simulink model "Excavator_Param_BOFTOF_Setup"  (R2026a)
settings: Solver=ode45  StopTime=0.2  AbsTol=1e-3  EnableMultiTasking=on
InitFcn:
  | if(~exist('ExcvLocal'))
  | ExcvGlobal = Excavator_Pin_Locations_global('Design A');
  | ExcvLocal  = Excavator_Pin_Locations_global2local(ExcvGlobal);
  | disp('Loading default pin locations...');
  | end
undefined symbols (not defined in the file or in its folder): A1, A2, B1, B2, B3, BOFTOF_boomAngle, BOFTOF_bucketAngle, BOFTOF_stickAngle, C1, C2, C3, C4, D1, D2, excv_data, X, Y, Z
libraries: nesl_utility x36, sm_lib x29, Excavator_Parts_Param_Lib x8, Linkage_Assembly_Lib x3, Arrowhead_Lib x3
(part 1 of 2)
Description:
  | Copyright 2022-2026 The MathWorks, Inc.
settings Model: Creator=smiller  LastModifiedBy=smiller
settings SimscapeCC: SimscapeNominalValues="[{\"value\":\"1\",\"unit\":\"A\"},{\"value\":\"1\",\"unit\":\"bar\"},{\"value\":\"1\",\"unit\":\"cm^2\"},{\"value\":\"1\",\"unit\":\"cm^3/s\"},{\"value\":\"1\",\"unit\":\"kJ/kg\"},{\"value\":\"1\",\"unit\":\"kW\"},{\"value\":\"1\",\"unit\":\"l\"},{\"value\":\"1\",\"unit\":\"N\"},{\"value\":\"1\",\"unit\":\"N*m\"},{\"value\":\"1\",\"unit\":\"V\"}]"  SimscapeLogSimulationStatistics=on
settings DiagnosticsConfigSet: SimMechanicsConflictingReferenceFrames=none  SimMechanicsUnsatisfiedHighPriorityTargets=none
settings ExplorerConfigSet: InternalSimMechanicsExplorerSettings="<ExplorerConfiguration><canonicalview>default</canonicalview><AnimationSetting><BasePlaybackSpeed>1.0</BasePlaybackSpeed><PlaybackSpeedFactor>1.0</PlaybackSpeedFactor></AnimationSetting><TilePanel><TileInfo><Tiles Columns=\"1\" Count=\"1\" Rows=\"1\"><Column Weight=\"1\"/><Row Weight=\"1\"/><Tile Height=\"1\" Width=\"1\" X=\"0\" Y=\"0\"/></Tiles></TileInfo><SceneInfo><SceneViewer><BGColor><R>1</R><G>1</G><B>1</B></BGColor><Camera><DoPerspective>off</DoPerspective><Position><X>6.08452747440039499</X><Y>2.23982062543228677</Y><Z>6.37263332562871465</Z></Position><Center><X>6.08452747440039499</X><Y>2.23982062543228677</Y><Z>-1.95928139490320063e-07</Z></Center><Up><X>0</X><Y>1</Y><Z>-0</Z></Up><ViewLimDist>1</ViewLimDist><YLim>4.12210355497723135</YLim><XLim>6.50790764061927973</XLim></Camera></SceneViewer></SceneInfo></TilePanel><MechEditorPanel><Cameras/><GfxPanelCameraMap/><VideoCreator><PlaybackSpeedRatio>1.0</PlaybackSpeedRatio><FrameRate>30</FrameRate><VideoFormat>Motion JPEG AVI</VideoFormat><FrameSize>auto</FrameSize></VideoCreator></MechEditorPanel></ExplorerConfiguration>"

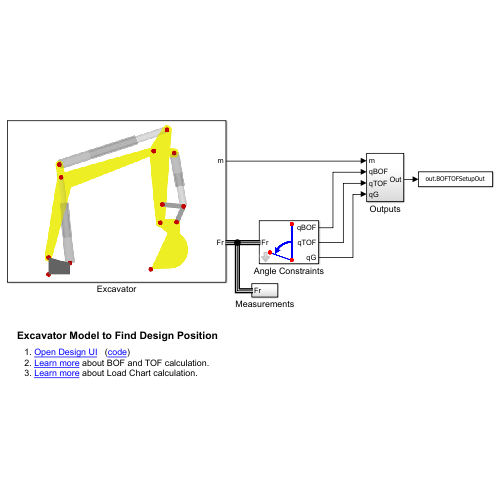
[thumbnail: Simulink's stored preview of the top-level diagram]
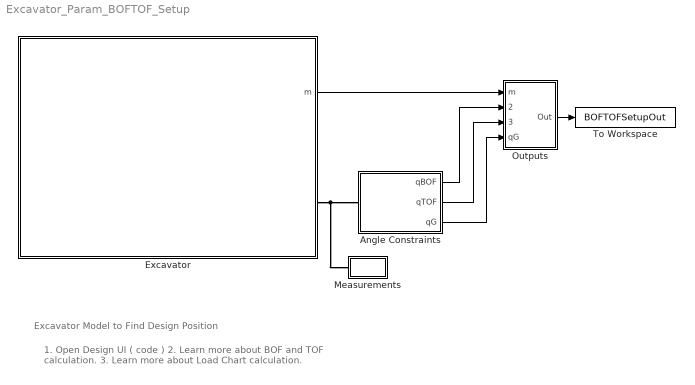
== system Excavator_Param_BOFTOF_Setup ==
  note: Excavator Model to Find Design Position
  note: 1. Open Design UI ( code )
      | 2. Learn more about BOF and TOF calculation.
      | 3. Learn more about Load Chart calculation.
  Angle Constraints : Subsystem  mask{target_angle_boom=BOFTOF_boomAngle, target_angle_stick=BOFTOF_stickAngle, target_angle_bucket=BOFTOF_bucketAngle, bar_opc=0.25, bar_dim=[2000 60 400], bar_clr=[0 0 1], checkbox_show_arc=on, arc_rad=1, arc_opc=0.25, arc_irs=0.75, arc_dep=1, arc_clr=[0 0 1]}
      mask prompts: target_angle_boom "Boom Target Angle (deg)"; target_angle_stick "Stick Target Angle (deg)"; target_angle_bucket "Bucket Target Angle (deg)"; bar_opc "Bar Opacity (0-1)"; bar_dim "Bar Dimensions [len wid depth] (m)"; bar_clr "Bar Color (0-1) [R G B]"; checkbox_show_arc "Show Arc"; arc_rad "Arc Outer Radius (m)"; arc_opc "Arc Opacity (0-1)"; arc_irs "Arc Inner Radius Scale (0-1)"; arc_dep "Arc Depth"; arc_clr "Arc Color (0-1) [R G B]"
      mask TypeOptions target_angle_boom: Boom Angle/target_angle
      mask TypeOptions target_angle_stick: Stick Angle/target_angle
      mask TypeOptions target_angle_bucket: Bucket Angle/target_angle
      mask TypeOptions bar_opc: Boom Angle/bar_opc | Bucket Angle/bar_opc | Stick Angle/bar_opc
      mask TypeOptions bar_dim: Boom Angle/bar_dim | Bucket Angle/bar_dim | Stick Angle/bar_dim
      mask TypeOptions bar_clr: Boom Angle/bar_clr | Bucket Angle/bar_clr | Stick Angle/bar_clr
      mask TypeOptions checkbox_show_arc: Boom Angle/checkbox_show_arc | Bucket Angle/checkbox_show_arc | Stick Angle/checkbox_show_arc
      mask TypeOptions arc_rad: Boom Angle/arc_rad | Bucket Angle/arc_rad | Stick Angle/arc_rad
      mask TypeOptions arc_opc: Boom Angle/arc_opc | Bucket Angle/arc_opc | Stick Angle/arc_opc
      mask TypeOptions arc_irs: Boom Angle/arc_irs | Bucket Angle/arc_irs | Stick Angle/arc_irs
      mask TypeOptions arc_dep: Boom Angle/arc_dep | Bucket Angle/arc_dep | Stick Angle/arc_dep
      mask TypeOptions arc_clr: Boom Angle/arc_clr | Bucket Angle/arc_clr | Stick Angle/arc_clr
      mask DialogControl Container3 Prompt: Appearance
      mask Display: image('Angle_Tools_IMAGE.png')
  Excavator : Subsystem
      mask Display: image('Excavator_Param_Full_IMAGE.png');
  Measurements : Subsystem
  Outputs : Subsystem
  To Workspace : ToWorkspace  VariableName=BOFTOFSetupOut  SaveFormat=Timeseries  SampleTime=-1
  wires:
  Outputs/1(Out) -> To Workspace/1
  Angle Constraints/1(qBOF) -> Outputs/2(qBOF)
  Angle Constraints/2(qTOF) -> Outputs/3(qTOF)
  Excavator/1(m) -> Outputs/1(m)
  Angle Constraints/3(qG) -> Outputs/4(qG)
  connections:
  Excavator/RConn1 -- Measurements/LConn1 -- Angle Constraints/LConn1

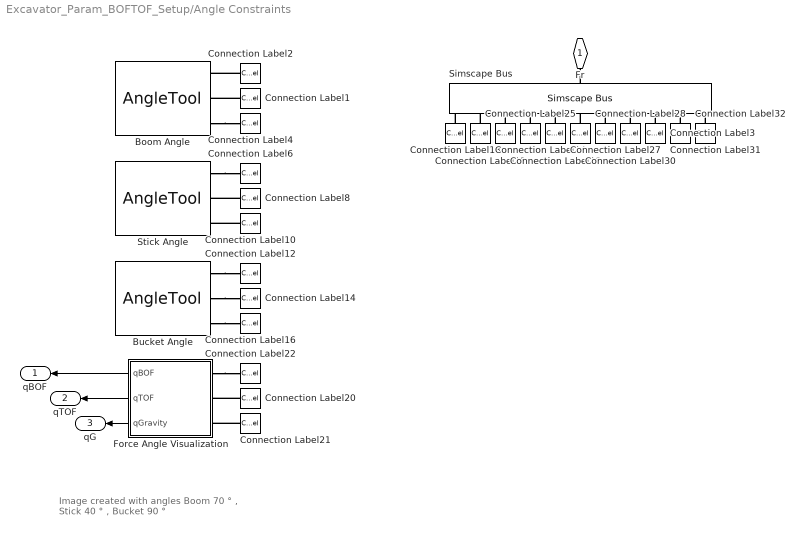
== system Excavator_Param_BOFTOF_Setup/Angle Constraints ==
  note: Image created with angles
      | Boom 70 ° , Stick 40 ° , Bucket 90 °
  Boom Angle : Linkage_Assembly_Lib/AngleTool  target_angle=target_angle_boom  checkbox_show_arc=on  arc_irs=arc_irs  arc_dep=arc_dep  arc_rad=arc_rad  arc_opc=arc_opc  arc_clr=arc_clr  bar_dim=bar_dim  bar_opc=bar_opc  bar_clr=bar_clr
  Bucket Angle : Linkage_Assembly_Lib/AngleTool  target_angle=target_angle_bucket  checkbox_show_arc=on  arc_irs=arc_irs  arc_dep=arc_dep  arc_rad=arc_rad  arc_opc=arc_opc  arc_clr=arc_clr  bar_dim=bar_dim  bar_opc=bar_opc  bar_clr=bar_clr
  Connection Label1 : ConnectionLabel  Label=A1
  Connection Label10 : ConnectionLabel  Label=B2
  Connection Label12 : ConnectionLabel  Label=D1
  Connection Label14 : ConnectionLabel  Label=C4
  Connection Label16 : ConnectionLabel  Label=C2
  Connection Label18 : ConnectionLabel  Label=A1
  Connection Label19 : ConnectionLabel  Label=A2
  Connection Label2 : ConnectionLabel  Label=A2
  Connection Label20 : ConnectionLabel  Label=C4
  Connection Label21 : ConnectionLabel  Label=B3
  Connection Label22 : ConnectionLabel  Label=D2
  Connection Label24 : ConnectionLabel  Label=B1
  Connection Label25 : ConnectionLabel  Label=B2
  Connection Label26 : ConnectionLabel  Label=B3
  Connection Label27 : ConnectionLabel  Label=C1
  Connection Label28 : ConnectionLabel  Label=C2
  Connection Label3 : ConnectionLabel  Label=C4
  Connection Label30 : ConnectionLabel  Label=C3
  Connection Label31 : ConnectionLabel  Label=D1
  Connection Label32 : ConnectionLabel  Label=D2
  Connection Label4 : ConnectionLabel  Label=B1
  Connection Label6 : ConnectionLabel  Label=C1
  Connection Label8 : ConnectionLabel  Label=B3
  Force Angle Visualization : Subsystem
      mask Display: image('Arrow_with_Reference_Line_IMAGE.png')
  Simscape Bus : SimscapeBus  HierarchyStrings=A1;A2;B1;B2;B3;C1;C2;C3;C4;D1;D2
  Stick Angle : Linkage_Assembly_Lib/AngleTool  target_angle=target_angle_stick  checkbox_show_arc=on  arc_irs=arc_irs  arc_dep=arc_dep  arc_rad=arc_rad  arc_opc=arc_opc  arc_clr=arc_clr  bar_dim=bar_dim  bar_opc=bar_opc  bar_clr=bar_clr
  Fr : PMIOPort  Side=Left
  qBOF : Outport
  qTOF : Outport  Port=2
  qG : Outport  Port=3
  wires:
  Force Angle Visualization/2(qTOF) -> qTOF/1
  Force Angle Visualization/1(qBOF) -> qBOF/1
  Force Angle Visualization/3(qGravity) -> qG/1
  connections:
  Connection Label10/LConn1 -- Stick Angle/LConn3
  Bucket Angle/LConn1 -- Connection Label12/LConn1
  Stick Angle/LConn1 -- Connection Label6/LConn1
  Boom Angle/LConn3 -- Connection Label4/LConn1
  Connection Label1/LConn1 -- Boom Angle/LConn2
  Connection Label21/LConn1 -- Force Angle Visualization/LConn3
  Connection Label2/LConn1 -- Boom Angle/LConn1
  Simscape Bus/RConn1 -- Fr/RConn1
  Connection Label8/LConn1 -- Stick Angle/LConn2
  Bucket Angle/LConn3 -- Connection Label16/LConn1
  Bucket Angle/LConn2 -- Connection Label14/LConn1
  Force Angle Visualization/LConn1 -- Connection Label22/LConn1
  Connection Label20/LConn1 -- Force Angle Visualization/LConn2
  Connection Label31/LConn1 -- Simscape Bus/LConn10
  Connection Label24/LConn1 -- Simscape Bus/LConn3
  Connection Label27/LConn1 -- Simscape Bus/LConn6
  Connection Label28/LConn1 -- Simscape Bus/LConn7
  Connection Label25/LConn1 -- Simscape Bus/LConn4
  Connection Label32/LConn1 -- Simscape Bus/LConn11
  Connection Label3/LConn1 -- Simscape Bus/LConn9
  Connection Label30/LConn1 -- Simscape Bus/LConn8
  Connection Label19/LConn1 -- Simscape Bus/LConn2
  Connection Label26/LConn1 -- Simscape Bus/LConn5
  Connection Label18/LConn1 -- Simscape Bus/LConn1

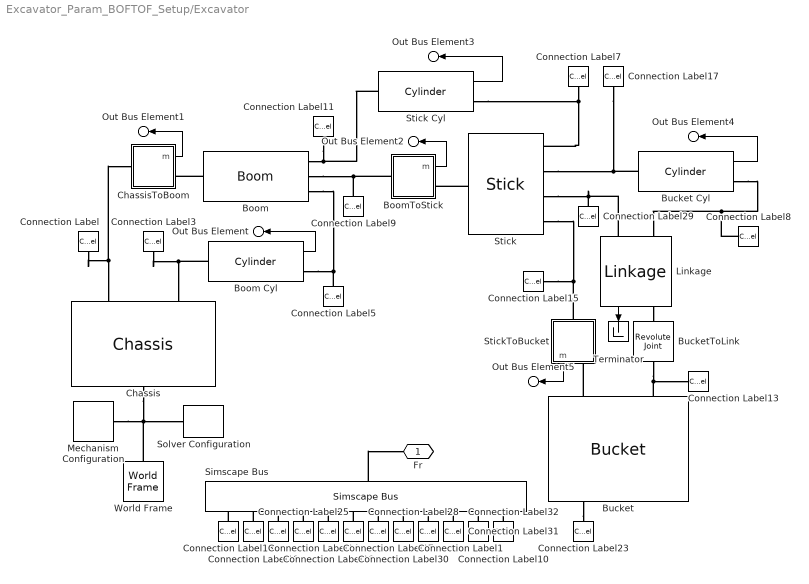
== system Excavator_Param_BOFTOF_Setup/Excavator ==
  Boom : Excavator_Parts_Param_Lib/Boom  part_thk=excv_data.arm.thk*1.05  part_clr=excv_data.arm.clr  opc=excv_data.arm.opc  pin_len=excv_data.pin.len  pin_rad=excv_data.pin.rad  pin_clr=excv_data.pin.clr  pin_opc=excv_data.pin.opc  Boom=ExcvLocal.Boom  part_mass=LoadChart_BoomMass
  Boom Cyl : Excavator_Parts_Param_Lib/Cylinder  cyl_clr=excv_data.cyl.clr  cyl_rad=excv_data.cyl.rad  cyl_opc=excv_data.cyl.opc  cyl_len=excv_data.boomcyl.len  pist_clr=excv_data.pist.clr  pist_rad=excv_data.pist.rad  pist_opc=excv_data.pist.opc  pist_len=excv_data.boompist.len
  BoomToStick : Subsystem
      mask Display: image('Excavator_Revolute_IMAGE.png')
  Bucket : Excavator_Parts_Param_Lib/Bucket  part_thk=excv_data.bucket.thk  part_clr=excv_data.bucket.clr  opc=excv_data.arm.opc  pin_len=excv_data.pin.len  pin_rad=excv_data.pin.rad  pin_clr=excv_data.pin.clr  pin_opc=excv_data.pin.opc  Bucket=ExcvLocal.Bucket  part_mass=LoadChart_BucketMass
  Bucket Cyl : Excavator_Parts_Param_Lib/Cylinder  cyl_clr=excv_data.cyl.clr  cyl_rad=excv_data.cyl.rad  cyl_opc=excv_data.cyl.opc  cyl_len=excv_data.bucketcyl.len  pist_clr=excv_data.pist.clr  pist_rad=excv_data.pist.rad  pist_opc=excv_data.pist.opc  pist_len=excv_data.bucketpist.len
  BucketToLink : sm_lib/Joints/Revolute Joint  JointMode=Normal  CompositeWrenchDir=FollowerOnBase  CompositeWrenchFrame=BaseFrame  SenseConstraintForce=off  SenseConstraintTorque=off  SenseTotalForce=off  SenseTotalTorque=off  PositionTargetSpecify=off  PositionTargetPriority=Low  PositionTargetValue=0  PositionTargetValueUnits=deg  VelocityTargetSpecify=off  VelocityTargetPriority=High  VelocityTargetValue=0  VelocityTargetValueUnits=deg/s  EquilibriumPosition=0  EquilibriumPositionUnits=deg  SpringStiffness=0  SpringStiffnessUnits=N*m/deg  DampingCoefficient=0  DampingCoefficientUnits=N*m/(deg/s)  LowerLimitSpecify=off  LowerLimitBound=-90  LowerLimitBoundUnits=deg  LowerLimitStiffness=1e4  LowerLimitStiffnessUnits=N*m/deg  LowerLimitDamping=10  LowerLimitDampingUnits=N*m/(deg/s)  LowerLimitTransitionRegionWidth=0.1  LowerLimitTransitionRegionWidthUnits=deg  UpperLimitSpecify=off  UpperLimitBound=90  UpperLimitBoundUnits=deg  UpperLimitStiffness=1e4  UpperLimitStiffnessUnits=N*m/deg  UpperLimitDamping=10  UpperLimitDampingUnits=N*m/(deg/s)  UpperLimitTransitionRegionWidth=0.1  UpperLimitTransitionRegionWidthUnits=deg  TorqueActuationMode=NoTorque  MotionActuationMode=ComputedMotion  SensePosition=off  SenseVelocity=off  SenseAcceleration=off  SenseTorqueForce=off  SenseLowerLimitTorqueForce=off  SenseUpperLimitTorqueForce=off
  Chassis : Excavator_Parts_Param_Lib/Chassis  Chassis=ExcvLocal.Chassis  opc=0  part_thk=excv_data.chassis.thk  part_clr=excv_data.chassis.clr  pin_clr=excv_data.pin.clr  pin_rad=excv_data.pin.rad  pin_len=excv_data.pin.len  pin_opc=excv_data.pin.opc
  ChassisToBoom : Subsystem
      mask Display: image('Excavator_Revolute_IMAGE.png')
  Connection Label : ConnectionLabel  Label=A1
  Connection Label1 : ConnectionLabel  Label=C4
  Connection Label10 : ConnectionLabel  Label=E1
  Connection Label11 : ConnectionLabel  Label=B2
  Connection Label13 : ConnectionLabel  Label=D1
  Connection Label15 : ConnectionLabel  Label=C4
  Connection Label17 : ConnectionLabel  Label=C2
  Connection Label18 : ConnectionLabel  Label=A1
  Connection Label19 : ConnectionLabel  Label=A2
  Connection Label23 : ConnectionLabel  Label=D2
  Connection Label24 : ConnectionLabel  Label=B1
  Connection Label25 : ConnectionLabel  Label=B2
  Connection Label26 : ConnectionLabel  Label=B3
  Connection Label27 : ConnectionLabel  Label=C1
  Connection Label28 : ConnectionLabel  Label=C2
  Connection Label29 : ConnectionLabel  Label=C3
  Connection Label3 : ConnectionLabel  Label=A2
  Connection Label30 : ConnectionLabel  Label=C3
  Connection Label31 : ConnectionLabel  Label=D1
  Connection Label32 : ConnectionLabel  Label=D2
  Connection Label5 : ConnectionLabel  Label=B1
  Connection Label7 : ConnectionLabel  Label=C1
  Connection Label8 : ConnectionLabel  Label=E1
  Connection Label9 : ConnectionLabel  Label=B3
  Linkage : Excavator_Parts_Param_Lib/Linkage  Linkage=ExcvLocal.Linkage  link_clr=excv_data.link.clr  link_thk=excv_data.link.thk  opc=excv_data.link.opc  pin_clr=excv_data.pin.clr  pin_rad=excv_data.pin.rad  pin_len=excv_data.pin.len  pin_opc=excv_data.pin.opc
  Mechanism Configuration : sm_lib/Utilities/Mechanism Configuration  UniformGravity=Constant  GravityVector=[0 -9.80665 0]  GravityVectorUnits=m/s^2  LinearizationDelta=0.001  JointModeTransitionNonlinearIterations=2
  Simscape Bus : SimscapeBus  HierarchyStrings=A1;A2;B1;B2;B3;C1;C2;C3;C4;D1;D2;E1
  Solver Configuration : nesl_utility/Solver Configuration  PhysicalDomain=network_engine_domain  SubClassName=solver  LeftPortType=input  RightPortType=generic  Tones=[]  Harmonics=[]  SimulateNoise=off  Profile=off  UseLocalSampling=off  EnableSwitchedLinearOptims=on  FrequencyDomain=off  UseCCode=off  RelTol=0.001  AbsTol=1e-06  MinStep=1e-09  ToWorkspace=off  RevertToSquareIcSolve=off  NumHomotopyIterations=100  PhasorMode=off  PhasorModeNumHarmonics=1  ConsistencySolver=NEWTON_FTOL  CanonicalOrdering=UNORDERED  OptimizeIntermediates=UNOPTIMIZED  IndexReductionMethod=DerivativeReplacement  DoDC=off  ResidualTolerance=1e-09  ConsistencyTolSource=GLOBAL  ConsistencyAbsTol=0.001  ConsistencyRelTol=0.001  ConsistencyTolFactor=0.001  UseLocalSolver=off  LocalSolverChoice=NE_BACKWARD_EULER_ADVANCER  ResolveIndetEquations=on  FunctionEvalNumThread=1  LocalSolverSampleTime=0.001  DoFixedCost=off  MaxNonlinIter=3  MaxModeIter=2  ComputeImpulses=off  ImpulseIterations=2  LinearAlgebra=Sparse  LinearAlgebraNumThread=0  EquationFormulation=NE_TIME_EF  DelaysMemoryBudget=1024  AutomaticFiltering=on  FilteringTimeConstant=0.001  PartitionStorageMethod=AS_NEEDED  PartitionMemoryBudget=1024  PartitionMethod=FAST  MultibodyUseLocalSolver=off  MultibodyLocalSolverChoice=ODE1  MultibodyLocalSolverSampleTime=0.001
  Stick : Excavator_Parts_Param_Lib/Stick  part_thk=excv_data.arm.thk  part_clr=excv_data.arm.clr*0.9  opc=excv_data.arm.opc  pin_len=excv_data.pin.len  pin_rad=excv_data.pin.rad  pin_opc=excv_data.pin.opc  pin_clr=excv_data.pin.clr  Stick=ExcvLocal.Stick  part_mass=LoadChart_StickMass
  Stick Cyl : Excavator_Parts_Param_Lib/Cylinder  cyl_clr=excv_data.cyl.clr  cyl_rad=excv_data.cyl.rad  cyl_opc=excv_data.cyl.opc  cyl_len=excv_data.stickcyl.len  pist_clr=excv_data.pist.clr  pist_rad=excv_data.pist.rad  pist_opc=excv_data.pist.opc  pist_len=excv_data.stickpist.len
  StickToBucket : Subsystem
      mask Display: image('Excavator_Revolute_IMAGE.png')
  Terminator : Terminator
  World Frame : sm_lib/Frames and Transforms/World Frame
  Fr : PMIOPort  Side=Right
  Out Bus Element : Outport  PortName=m  Element=cBoomL
  Out Bus Element3 : Outport  PortName=m  Element=cStick
  Out Bus Element4 : Outport  PortName=m  Element=cBucket
  Out Bus Element1 : Outport  PortName=m  Element=jC2B
  Out Bus Element2 : Outport  PortName=m  Element=jB2S
  Out Bus Element5 : Outport  PortName=m  Element=jS2B
  wires:
  Boom Cyl/1 -> Out Bus Element/1
  Stick Cyl/1 -> Out Bus Element3/1
  Bucket Cyl/1 -> Out Bus Element4/1
  ChassisToBoom/1(m) -> Out Bus Element1/1
  BoomToStick/1(m) -> Out Bus Element2/1
  StickToBucket/1(m) -> Out Bus Element5/1
  Linkage/1 -> Terminator/1
  connections:
  Connection Label/LConn1 -- Chassis/RConn1 -- ChassisToBoom/LConn1
  Connection Label29/LConn1 -- Stick/RConn3 -- Linkage/LConn1
  Connection Label7/LConn1 -- Stick Cyl/RConn1 -- Stick/RConn1
  Connection Label11/LConn1 -- Boom/RConn1 -- Stick Cyl/LConn1
  Bucket/LConn1 -- StickToBucket/RConn1
  Connection Label5/LConn1 -- Boom Cyl/RConn1 -- Boom/RConn3
  World Frame/RConn1 -- Chassis/LConn1 -- Solver Configuration/RConn1 -- Mechanism Configuration/RConn1
  BucketToLink/LConn1 -- Bucket/LConn2 -- Connection Label13/LConn1
  Connection Label17/LConn1 -- Bucket Cyl/LConn1 -- Stick/RConn2
  Simscape Bus/RConn1 -- Fr/RConn1
  Connection Label3/LConn1 -- Boom Cyl/LConn1 -- Chassis/RConn2
  Boom/LConn1 -- ChassisToBoom/RConn1
  Connection Label9/LConn1 -- Boom/RConn2 -- BoomToStick/LConn1
  Stick/LConn1 -- BoomToStick/RConn1
  StickToBucket/LConn1 -- Stick/RConn4 -- Connection Label15/LConn1
  Bucket/RConn1 -- Connection Label23/LConn1
  Bucket Cyl/RConn1 -- Connection Label8/LConn1 -- Linkage/LConn2
  Linkage/RConn1 -- BucketToLink/RConn1
  Connection Label26/LConn1 -- Simscape Bus/LConn5
  Connection Label25/LConn1 -- Simscape Bus/LConn4
  Connection Label28/LConn1 -- Simscape Bus/LConn7
  Connection Label24/LConn1 -- Simscape Bus/LConn3
  Connection Label31/LConn1 -- Simscape Bus/LConn10
  Connection Label1/LConn1 -- Simscape Bus/LConn9
  Connection Label19/LConn1 -- Simscape Bus/LConn2
  Connection Label30/LConn1 -- Simscape Bus/LConn8
  Connection Label27/LConn1 -- Simscape Bus/LConn6
  Connection Label18/LConn1 -- Simscape Bus/LConn1
  Connection Label32/LConn1 -- Simscape Bus/LConn11
  Connection Label10/LConn1 -- Simscape Bus/LConn12

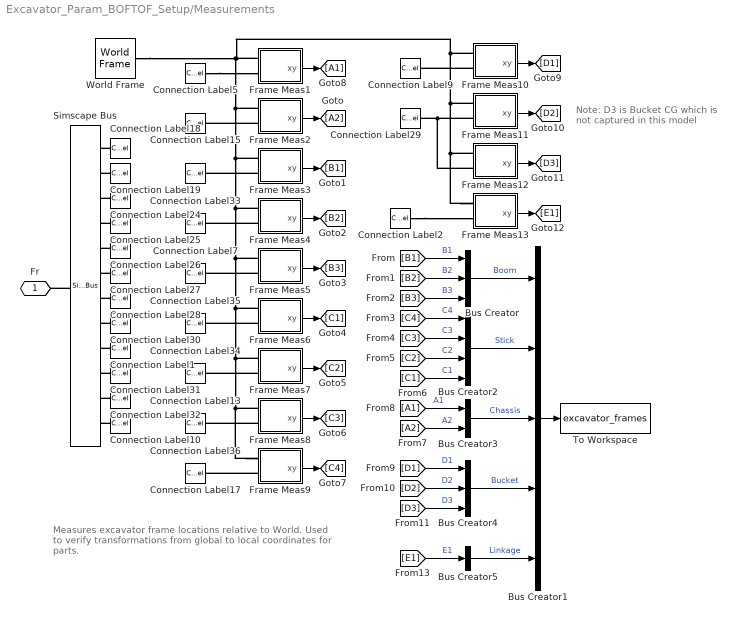
== system Excavator_Param_BOFTOF_Setup/Measurements ==
  note: Measures excavator frame locations relative to World. Used to verify transformations from global to local coordinates for parts.
  note: Note: D3 is Bucket CG which is not captured in this model
  Bus Creator : BusCreator  Inputs=3
  Bus Creator1 : BusCreator  Inputs=5
  Bus Creator2 : BusCreator  Inputs=4
  Bus Creator3 : BusCreator  Inputs=2
  Bus Creator4 : BusCreator  Inputs=3
  Bus Creator5 : BusCreator  Inputs=1
  Connection Label1 : ConnectionLabel  Label=C4
  Connection Label10 : ConnectionLabel  Label=E1
  Connection Label13 : ConnectionLabel  Label=C2
  Connection Label15 : ConnectionLabel  Label=A2
  Connection Label17 : ConnectionLabel  Label=C4
  Connection Label18 : ConnectionLabel  Label=A1
  Connection Label19 : ConnectionLabel  Label=A2
  Connection Label2 : ConnectionLabel  Label=E1
  Connection Label24 : ConnectionLabel  Label=B1
  Connection Label25 : ConnectionLabel  Label=B2
  Connection Label26 : ConnectionLabel  Label=B3
  Connection Label27 : ConnectionLabel  Label=C1
  Connection Label28 : ConnectionLabel  Label=C2
  Connection Label29 : ConnectionLabel  Label=D2
  Connection Label30 : ConnectionLabel  Label=C3
  Connection Label31 : ConnectionLabel  Label=D1
  Connection Label32 : ConnectionLabel  Label=D2
  Connection Label33 : ConnectionLabel  Label=B1
  Connection Label34 : ConnectionLabel  Label=C1
  Connection Label35 : ConnectionLabel  Label=B3
  Connection Label36 : ConnectionLabel  Label=C3
  Connection Label5 : ConnectionLabel  Label=A1
  Connection Label7 : ConnectionLabel  Label=B2
  Connection Label9 : ConnectionLabel  Label=D1
  Frame Meas1 : Subsystem
  Frame Meas10 : Subsystem
  Frame Meas11 : Subsystem
  Frame Meas12 : Subsystem
  Frame Meas13 : Subsystem
  Frame Meas2 : Subsystem
  Frame Meas3 : Subsystem
  Frame Meas4 : Subsystem
  Frame Meas5 : Subsystem
  Frame Meas6 : Subsystem
  Frame Meas7 : Subsystem
  Frame Meas8 : Subsystem
  Frame Meas9 : Subsystem
  Simscape Bus : SimscapeBus  HierarchyStrings=A1;A2;B1;B2;B3;C1;C2;C3;C4;D1;D2;E1
  To Workspace : ToWorkspace  VariableName=excavator_frames  SaveFormat=Timeseries  SampleTime=-1
      settings: MaxDataPoints=1
  World Frame : sm_lib/Frames and Transforms/World Frame
  Fr : PMIOPort  Side=Left
  wires:
  Frame Meas13/1(xy) -> [E1]
  [B3] -> Bus Creator/3  "B3"
  Frame Meas10/1(xy) -> [D1]
  Frame Meas9/1(xy) -> [C4]
  [A2] -> Bus Creator3/2  "A2"
  Frame Meas12/1(xy) -> [D3]
  Frame Meas2/1(xy) -> [A2]
  Frame Meas6/1(xy) -> [C1]
  [B2] -> Bus Creator/2  "B2"
  Frame Meas3/1(xy) -> [B1]
  Frame Meas5/1(xy) -> [B3]
  [C3] -> Bus Creator2/2  "C3"
  [A1] -> Bus Creator3/1  "A1"
  Frame Meas4/1(xy) -> [B2]
  Frame Meas1/1(xy) -> [A1]
  [D3] -> Bus Creator4/3  "D3"
  Bus Creator/1 -> Bus Creator1/1  "Boom"
  [B1] -> Bus Creator/1  "B1"
  Frame Meas8/1(xy) -> [C3]
  [D1] -> Bus Creator4/1  "D1"
  Frame Meas11/1(xy) -> [D2]
  Frame Meas7/1(xy) -> [C2]
  Bus Creator3/1 -> Bus Creator1/3  "Chassis"
  [C1] -> Bus Creator2/4  "C1"
  [C2] -> Bus Creator2/3  "C2"
  Bus Creator4/1 -> Bus Creator1/4  "Bucket"
  [D2] -> Bus Creator4/2  "D2"
  Bus Creator2/1 -> Bus Creator1/2  "Stick"
  [E1] -> Bus Creator5/1  "E1"
  Bus Creator1/1 -> To Workspace/1
  [C4] -> Bus Creator2/1  "C4"
  Bus Creator5/1 -> Bus Creator1/5  "Linkage"
  connections:
  Frame Meas13/LConn1 -- Frame Meas12/LConn1 -- Frame Meas11/LConn1 -- Frame Meas10/LConn1 -- Frame Meas1/LConn1 -- World Frame/RConn1 -- Frame Meas2/LConn1 -- Frame Meas3/LConn1 -- Frame Meas4/LConn1 -- Frame Meas5/LConn1 -- Frame Meas6/LConn1 -- Frame Meas9/LConn1 -- Frame Meas8/LConn1 -- Frame Meas7/LConn1
  Connection Label5/LConn1 -- Frame Meas1/LConn2
  Connection Label2/LConn1 -- Frame Meas13/LConn2
  Frame Meas10/LConn2 -- Connection Label9/LConn1
  Frame Meas7/LConn2 -- Connection Label13/LConn1
  Frame Meas9/LConn2 -- Connection Label17/LConn1
  Frame Meas8/LConn2 -- Connection Label36/LConn1
  Frame Meas4/LConn2 -- Connection Label7/LConn1
  Frame Meas11/LConn2 -- Frame Meas12/LConn2 -- Connection Label29/LConn1
  Frame Meas6/LConn2 -- Connection Label34/LConn1
  Frame Meas3/LConn2 -- Connection Label33/LConn1
  Frame Meas5/LConn2 -- Connection Label35/LConn1
  Frame Meas2/LConn2 -- Connection Label15/LConn1
  Simscape Bus/RConn1 -- Fr/RConn1
  Connection Label32/LConn1 -- Simscape Bus/LConn11
  Connection Label30/LConn1 -- Simscape Bus/LConn8
  Connection Label1/LConn1 -- Simscape Bus/LConn9
  Connection Label19/LConn1 -- Simscape Bus/LConn2
  Connection Label27/LConn1 -- Simscape Bus/LConn6
  Connection Label31/LConn1 -- Simscape Bus/LConn10
  Connection Label25/LConn1 -- Simscape Bus/LConn4
  Connection Label18/LConn1 -- Simscape Bus/LConn1
  Connection Label28/LConn1 -- Simscape Bus/LConn7
  Connection Label26/LConn1 -- Simscape Bus/LConn5
  Connection Label10/LConn1 -- Simscape Bus/LConn12
  Connection Label24/LConn1 -- Simscape Bus/LConn3

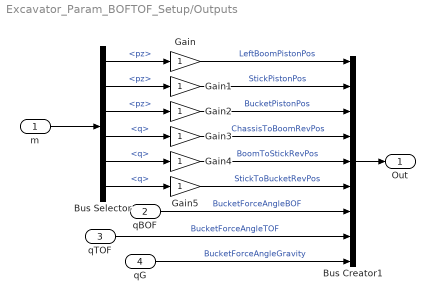
== system Excavator_Param_BOFTOF_Setup/Outputs ==
  m : Inport
  qBOF : Inport  Port=2
  qTOF : Inport  Port=3
  qG : Inport  Port=4
  Bus Creator1 : BusCreator  Inputs=9
  Bus Selector : BusSelector  OutputSignals=cBoomL.pz,cStick.pz,cBucket.pz,jC2B.q,jB2S.q,jS2B.q
  Gain{,1..5} (6 alike) : Gain
  Out : Outport
  wires:
  Gain5/1 -> Bus Creator1/6  "StickToBucketRevPos"
  Bus Selector/2 -> Gain1/1  "<pz>"
  Bus Selector/1 -> Gain/1  "<pz>"
  Gain1/1 -> Bus Creator1/2  "StickPistonPos"
  Bus Selector/4 -> Gain3/1  "<q>"
  Gain/1 -> Bus Creator1/1  "LeftBoomPistonPos"
  Bus Selector/5 -> Gain4/1  "<q>"
  Gain4/1 -> Bus Creator1/5  "BoomToStickRevPos"
  Bus Creator1/1 -> Out/1
  Bus Selector/6 -> Gain5/1  "<q>"
  Gain2/1 -> Bus Creator1/3  "BucketPistonPos"
  Gain3/1 -> Bus Creator1/4  "ChassisToBoomRevPos"
  Bus Selector/3 -> Gain2/1  "<pz>"
  qTOF/1 -> Bus Creator1/8  "BucketForceAngleTOF"
  m/1 -> Bus Selector/1
  qBOF/1 -> Bus Creator1/7  "BucketForceAngleBOF"
  qG/1 -> Bus Creator1/9  "BucketForceAngleGravity"

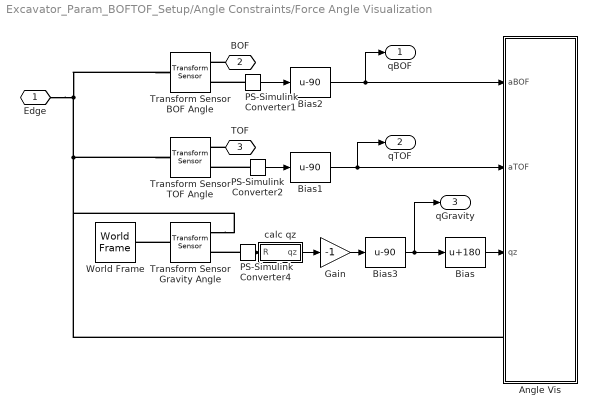
== system Excavator_Param_BOFTOF_Setup/Angle Constraints/Force Angle Visualization ==
  Angle Vis : Subsystem
  Bias : Bias  Bias=180  SaturateOnIntegerOverflow=off
  Bias1 : Bias  Bias=-90  SaturateOnIntegerOverflow=off
  Bias2 : Bias  Bias=-90  SaturateOnIntegerOverflow=off
  Bias3 : Bias  Bias=-90  SaturateOnIntegerOverflow=off
  Gain : Gain  Gain=-1
  PS-Simulink Converter1 : nesl_utility/PS-Simulink Converter  PhysicalDomain=network_engine_domain  SubClassName=ps_output  LeftPortType=input  RightPortType=output  PseudoPeriodic=off  Frequencies=[]  VectorFormat=inherit  Unit=deg  AffineConversion=off
  PS-Simulink Converter2 : nesl_utility/PS-Simulink Converter  PhysicalDomain=network_engine_domain  SubClassName=ps_output  LeftPortType=input  RightPortType=output  PseudoPeriodic=off  Frequencies=[]  VectorFormat=inherit  Unit=deg  AffineConversion=off
  PS-Simulink Converter4 : nesl_utility/PS-Simulink Converter  PhysicalDomain=network_engine_domain  SubClassName=ps_output  LeftPortType=input  RightPortType=output  PseudoPeriodic=off  Frequencies=[]  VectorFormat=inherit  Unit=1  AffineConversion=off
  Transform Sensor BOF Angle : sm_lib/Frames and Transforms/Transform Sensor  MeasurementFrame=Base  RotationSequence=XYX  SenseAngle=off  SenseAxis=off  SenseQ=off  SenseR=off  SenseRotationSequence=off  SenseOmegaX=off  SenseOmegaY=off  SenseOmegaZ=off  SenseOmega=off  SenseQDot=off  SenseRDot=off  SenseRotationSequenceDot=off  SenseAlphaX=off  SenseAlphaY=off  SenseAlphaZ=off  SenseAlpha=off  SenseQDDot=off  SenseRDDot=off  SenseX=off  SenseY=off  SenseZ=off  SenseXYZ=off  SenseRad=off  SenseAzim=on  SenseDist=off  SenseInc=off  SenseXDot=off  SenseYDot=off  SenseZDot=off  SenseXYZDot=off  SenseRadDot=off  SenseAzimDot=off  SenseDistDot=off  SenseIncDot=off  SenseXDDot=off  SenseYDDot=off  SenseZDDot=off  SenseXYZDDot=off  SenseRadDDot=off  SenseAzimDDot=off  SenseDistDDot=off  SenseIncDDot=off
  Transform Sensor Gravity Angle : sm_lib/Frames and Transforms/Transform Sensor  MeasurementFrame=World  RotationSequence=XYX  SenseAngle=off  SenseAxis=off  SenseQ=off  SenseR=on  SenseRotationSequence=off  SenseOmegaX=off  SenseOmegaY=off  SenseOmegaZ=off  SenseOmega=off  SenseQDot=off  SenseRDot=off  SenseRotationSequenceDot=off  SenseAlphaX=off  SenseAlphaY=off  SenseAlphaZ=off  SenseAlpha=off  SenseQDDot=off  SenseRDDot=off  SenseX=off  SenseY=off  SenseZ=off  SenseXYZ=off  SenseRad=off  SenseAzim=off  SenseDist=off  SenseInc=off  SenseXDot=off  SenseYDot=off  SenseZDot=off  SenseXYZDot=off  SenseRadDot=off  SenseAzimDot=off  SenseDistDot=off  SenseIncDot=off  SenseXDDot=off  SenseYDDot=off  SenseZDDot=off  SenseXYZDDot=off  SenseRadDDot=off  SenseAzimDDot=off  SenseDistDDot=off  SenseIncDDot=off
  Transform Sensor TOF Angle : sm_lib/Frames and Transforms/Transform Sensor  MeasurementFrame=Base  RotationSequence=XYX  SenseAngle=off  SenseAxis=off  SenseQ=off  SenseR=off  SenseRotationSequence=off  SenseOmegaX=off  SenseOmegaY=off  SenseOmegaZ=off  SenseOmega=off  SenseQDot=off  SenseRDot=off  SenseRotationSequenceDot=off  SenseAlphaX=off  SenseAlphaY=off  SenseAlphaZ=off  SenseAlpha=off  SenseQDDot=off  SenseRDDot=off  SenseX=off  SenseY=off  SenseZ=off  SenseXYZ=off  SenseRad=off  SenseAzim=on  SenseDist=off  SenseInc=off  SenseXDot=off  SenseYDot=off  SenseZDot=off  SenseXYZDot=off  SenseRadDot=off  SenseAzimDot=off  SenseDistDot=off  SenseIncDot=off  SenseXDDot=off  SenseYDDot=off  SenseZDDot=off  SenseXYZDDot=off  SenseRadDDot=off  SenseAzimDDot=off  SenseDistDDot=off  SenseIncDDot=off
  World Frame : sm_lib/Frames and Transforms/World Frame
  calc qz : Subsystem
  Edge : PMIOPort  Side=Left
  BOF : PMIOPort  Port=2  Side=Left
  TOF : PMIOPort  Port=3  Side=Left
  qBOF : Outport
  qTOF : Outport  Port=2
  qGravity : Outport  Port=3
  wires:
  PS-Simulink Converter2/1 -> Bias1/1
  PS-Simulink Converter1/1 -> Bias2/1
  PS-Simulink Converter4/1 -> calc qz/1(R)
  calc qz/1(qz) -> Gain/1
  Bias3/1 -> Bias/1, qGravity/1
  Bias/1 -> Angle Vis/3(qz)
  Bias1/1 -> qTOF/1, Angle Vis/2(aTOF)
  Bias2/1 -> Angle Vis/1(aBOF), qBOF/1
  Gain/1 -> Bias3/1
  connections:
  Edge/RConn1 -- Transform Sensor TOF Angle/LConn1 -- Transform Sensor Gravity Angle/RConn1 -- Angle Vis/LConn1 -- Transform Sensor BOF Angle/LConn1
  PS-Simulink Converter2/LConn1 -- Transform Sensor TOF Angle/RConn2
  BOF/RConn1 -- Transform Sensor BOF Angle/RConn1
  TOF/RConn1 -- Transform Sensor TOF Angle/RConn1
  PS-Simulink Converter1/LConn1 -- Transform Sensor BOF Angle/RConn2
  Transform Sensor Gravity Angle/LConn1 -- World Frame/RConn1
  PS-Simulink Converter4/LConn1 -- Transform Sensor Gravity Angle/RConn2

== system Excavator_Param_BOFTOF_Setup/Excavator/BoomToStick ==
  BoomToStick : sm_lib/Joints/Revolute Joint  JointMode=Normal  CompositeWrenchDir=FollowerOnBase  CompositeWrenchFrame=BaseFrame  SenseConstraintForce=off  SenseConstraintTorque=off  SenseTotalForce=off  SenseTotalTorque=off  PositionTargetSpecify=on  PositionTargetPriority=High  PositionTargetValue=0  PositionTargetValueUnits=deg  VelocityTargetSpecify=off  VelocityTargetPriority=High  VelocityTargetValue=0  VelocityTargetValueUnits=deg/s  EquilibriumPosition=0  EquilibriumPositionUnits=deg  SpringStiffness=0  SpringStiffnessUnits=N*m/deg  DampingCoefficient=0  DampingCoefficientUnits=N*m/(deg/s)  LowerLimitSpecify=off  LowerLimitBound=-90  LowerLimitBoundUnits=deg  LowerLimitStiffness=1e4  LowerLimitStiffnessUnits=N*m/deg  LowerLimitDamping=10  LowerLimitDampingUnits=N*m/(deg/s)  LowerLimitTransitionRegionWidth=0.1  LowerLimitTransitionRegionWidthUnits=deg  UpperLimitSpecify=off  UpperLimitBound=90  UpperLimitBoundUnits=deg  UpperLimitStiffness=1e4  UpperLimitStiffnessUnits=N*m/deg  UpperLimitDamping=10  UpperLimitDampingUnits=N*m/(deg/s)  UpperLimitTransitionRegionWidth=0.1  UpperLimitTransitionRegionWidthUnits=deg  TorqueActuationMode=NoTorque  MotionActuationMode=ComputedMotion  SensePosition=on  SenseVelocity=off  SenseAcceleration=off  SenseTorqueForce=off  SenseLowerLimitTorqueForce=off  SenseUpperLimitTorqueForce=off
  PS-Simulink Converter : nesl_utility/PS-Simulink Converter  PhysicalDomain=network_engine_domain  SubClassName=ps_output  LeftPortType=input  RightPortType=output  PseudoPeriodic=off  Frequencies=[]  VectorFormat=inherit  Unit=deg  AffineConversion=off
  B : PMIOPort  Side=Left
  F : PMIOPort  Port=2  Side=Right
  Out Bus Element6 : Outport  PortName=m  Element=q
  wires:
  PS-Simulink Converter/1 -> Out Bus Element6/1
  connections:
  BoomToStick/LConn1 -- B/RConn1
  PS-Simulink Converter/LConn1 -- BoomToStick/RConn2
  F/RConn1 -- BoomToStick/RConn1

== system Excavator_Param_BOFTOF_Setup/Excavator/ChassisToBoom ==
  ChassisToBoom : sm_lib/Joints/Revolute Joint  JointMode=Normal  CompositeWrenchDir=FollowerOnBase  CompositeWrenchFrame=BaseFrame  SenseConstraintForce=off  SenseConstraintTorque=off  SenseTotalForce=off  SenseTotalTorque=off  PositionTargetSpecify=on  PositionTargetPriority=High  PositionTargetValue=0  PositionTargetValueUnits=deg  VelocityTargetSpecify=off  VelocityTargetPriority=High  VelocityTargetValue=0  VelocityTargetValueUnits=deg/s  EquilibriumPosition=0  EquilibriumPositionUnits=deg  SpringStiffness=0  SpringStiffnessUnits=N*m/deg  DampingCoefficient=0  DampingCoefficientUnits=N*m/(deg/s)  LowerLimitSpecify=off  LowerLimitBound=-90  LowerLimitBoundUnits=deg  LowerLimitStiffness=1e4  LowerLimitStiffnessUnits=N*m/deg  LowerLimitDamping=10  LowerLimitDampingUnits=N*m/(deg/s)  LowerLimitTransitionRegionWidth=0.1  LowerLimitTransitionRegionWidthUnits=deg  UpperLimitSpecify=off  UpperLimitBound=90  UpperLimitBoundUnits=deg  UpperLimitStiffness=1e4  UpperLimitStiffnessUnits=N*m/deg  UpperLimitDamping=10  UpperLimitDampingUnits=N*m/(deg/s)  UpperLimitTransitionRegionWidth=0.1  UpperLimitTransitionRegionWidthUnits=deg  TorqueActuationMode=NoTorque  MotionActuationMode=ComputedMotion  SensePosition=on  SenseVelocity=off  SenseAcceleration=off  SenseTorqueForce=off  SenseLowerLimitTorqueForce=off  SenseUpperLimitTorqueForce=off
  PS-Simulink Converter : nesl_utility/PS-Simulink Converter  PhysicalDomain=network_engine_domain  SubClassName=ps_output  LeftPortType=input  RightPortType=output  PseudoPeriodic=off  Frequencies=[]  VectorFormat=inherit  Unit=deg  AffineConversion=off
  B : PMIOPort  Side=Left
  F : PMIOPort  Port=2  Side=Right
  Out Bus Element : Outport  PortName=m  Element=q
  wires:
  PS-Simulink Converter/1 -> Out Bus Element/1
  connections:
  PS-Simulink Converter/LConn1 -- ChassisToBoom/RConn2
  B/RConn1 -- ChassisToBoom/LConn1
  F/RConn1 -- ChassisToBoom/RConn1

== system Excavator_Param_BOFTOF_Setup/Excavator/StickToBucket ==
  PS-Simulink Converter : nesl_utility/PS-Simulink Converter  PhysicalDomain=network_engine_domain  SubClassName=ps_output  LeftPortType=input  RightPortType=output  PseudoPeriodic=off  Frequencies=[]  VectorFormat=inherit  Unit=deg  AffineConversion=off
  StickToBucket : sm_lib/Joints/Revolute Joint  JointMode=Normal  CompositeWrenchDir=FollowerOnBase  CompositeWrenchFrame=BaseFrame  SenseConstraintForce=off  SenseConstraintTorque=off  SenseTotalForce=off  SenseTotalTorque=off  PositionTargetSpecify=on  PositionTargetPriority=High  PositionTargetValue=0  PositionTargetValueUnits=deg  VelocityTargetSpecify=off  VelocityTargetPriority=High  VelocityTargetValue=0  VelocityTargetValueUnits=deg/s  EquilibriumPosition=0  EquilibriumPositionUnits=deg  SpringStiffness=0  SpringStiffnessUnits=N*m/deg  DampingCoefficient=0  DampingCoefficientUnits=N*m/(deg/s)  LowerLimitSpecify=off  LowerLimitBound=-90  LowerLimitBoundUnits=deg  LowerLimitStiffness=1e4  LowerLimitStiffnessUnits=N*m/deg  LowerLimitDamping=10  LowerLimitDampingUnits=N*m/(deg/s)  LowerLimitTransitionRegionWidth=0.1  LowerLimitTransitionRegionWidthUnits=deg  UpperLimitSpecify=off  UpperLimitBound=90  UpperLimitBoundUnits=deg  UpperLimitStiffness=1e4  UpperLimitStiffnessUnits=N*m/deg  UpperLimitDamping=10  UpperLimitDampingUnits=N*m/(deg/s)  UpperLimitTransitionRegionWidth=0.1  UpperLimitTransitionRegionWidthUnits=deg  TorqueActuationMode=NoTorque  MotionActuationMode=ComputedMotion  SensePosition=on  SenseVelocity=off  SenseAcceleration=off  SenseTorqueForce=off  SenseLowerLimitTorqueForce=off  SenseUpperLimitTorqueForce=off
  B : PMIOPort  Side=Left
  F : PMIOPort  Port=2  Side=Right
  Out Bus Element : Outport  PortName=m  Element=q
  wires:
  PS-Simulink Converter/1 -> Out Bus Element/1
  connections:
  F/RConn1 -- StickToBucket/RConn1
  StickToBucket/LConn1 -- B/RConn1
  PS-Simulink Converter/LConn1 -- StickToBucket/RConn2

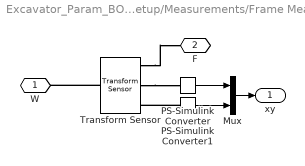
== system Excavator_Param_BOFTOF_Setup/Measurements/Frame Meas1 ==
  Mux : Mux  Inputs=2
  PS-Simulink Converter : nesl_utility/PS-Simulink Converter  PhysicalDomain=network_engine_domain  SubClassName=ps_output  LeftPortType=input  RightPortType=output  PseudoPeriodic=off  Frequencies=[]  VectorFormat=inherit  Unit=inherit  AffineConversion=off
  PS-Simulink Converter1 : nesl_utility/PS-Simulink Converter  PhysicalDomain=network_engine_domain  SubClassName=ps_output  LeftPortType=input  RightPortType=output  PseudoPeriodic=off  Frequencies=[]  VectorFormat=inherit  Unit=inherit  AffineConversion=off
  Transform Sensor : sm_lib/Frames and Transforms/Transform Sensor  MeasurementFrame=World  RotationSequence=XYX  SenseAngle=off  SenseAxis=off  SenseQ=off  SenseR=off  SenseRotationSequence=off  SenseOmegaX=off  SenseOmegaY=off  SenseOmegaZ=off  SenseOmega=off  SenseQDot=off  SenseRDot=off  SenseRotationSequenceDot=off  SenseAlphaX=off  SenseAlphaY=off  SenseAlphaZ=off  SenseAlpha=off  SenseQDDot=off  SenseRDDot=off  SenseX=on  SenseY=on  SenseZ=off  SenseXYZ=off  SenseRad=off  SenseAzim=off  SenseDist=off  SenseInc=off  SenseXDot=off  SenseYDot=off  SenseZDot=off  SenseXYZDot=off  SenseRadDot=off  SenseAzimDot=off  SenseDistDot=off  SenseIncDot=off  SenseXDDot=off  SenseYDDot=off  SenseZDDot=off  SenseXYZDDot=off  SenseRadDDot=off  SenseAzimDDot=off  SenseDistDDot=off  SenseIncDDot=off
  W : PMIOPort  Side=Left
  F : PMIOPort  Port=2  Side=Left
  xy : Outport
  wires:
  PS-Simulink Converter1/1 -> Mux/2
  PS-Simulink Converter/1 -> Mux/1
  Mux/1 -> xy/1
  connections:
  Transform Sensor/LConn1 -- W/RConn1
  Transform Sensor/RConn2 -- PS-Simulink Converter/LConn1
  PS-Simulink Converter1/LConn1 -- Transform Sensor/RConn3
  Transform Sensor/RConn1 -- F/RConn1

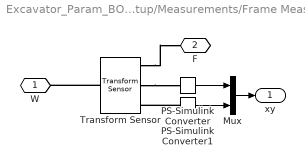
== system Excavator_Param_BOFTOF_Setup/Measurements/Frame Meas10 ==
  Mux : Mux  Inputs=2
  PS-Simulink Converter : nesl_utility/PS-Simulink Converter  PhysicalDomain=network_engine_domain  SubClassName=ps_output  LeftPortType=input  RightPortType=output  PseudoPeriodic=off  Frequencies=[]  VectorFormat=inherit  Unit=inherit  AffineConversion=off
  PS-Simulink Converter1 : nesl_utility/PS-Simulink Converter  PhysicalDomain=network_engine_domain  SubClassName=ps_output  LeftPortType=input  RightPortType=output  PseudoPeriodic=off  Frequencies=[]  VectorFormat=inherit  Unit=inherit  AffineConversion=off
  Transform Sensor : sm_lib/Frames and Transforms/Transform Sensor  MeasurementFrame=World  RotationSequence=XYX  SenseAngle=off  SenseAxis=off  SenseQ=off  SenseR=off  SenseRotationSequence=off  SenseOmegaX=off  SenseOmegaY=off  SenseOmegaZ=off  SenseOmega=off  SenseQDot=off  SenseRDot=off  SenseRotationSequenceDot=off  SenseAlphaX=off  SenseAlphaY=off  SenseAlphaZ=off  SenseAlpha=off  SenseQDDot=off  SenseRDDot=off  SenseX=on  SenseY=on  SenseZ=off  SenseXYZ=off  SenseRad=off  SenseAzim=off  SenseDist=off  SenseInc=off  SenseXDot=off  SenseYDot=off  SenseZDot=off  SenseXYZDot=off  SenseRadDot=off  SenseAzimDot=off  SenseDistDot=off  SenseIncDot=off  SenseXDDot=off  SenseYDDot=off  SenseZDDot=off  SenseXYZDDot=off  SenseRadDDot=off  SenseAzimDDot=off  SenseDistDDot=off  SenseIncDDot=off
  W : PMIOPort  Side=Left
  F : PMIOPort  Port=2  Side=Left
  xy : Outport
  wires:
  Mux/1 -> xy/1
  PS-Simulink Converter/1 -> Mux/1
  PS-Simulink Converter1/1 -> Mux/2
  connections:
  Transform Sensor/RConn1 -- F/RConn1
  PS-Simulink Converter1/LConn1 -- Transform Sensor/RConn3
  Transform Sensor/RConn2 -- PS-Simulink Converter/LConn1
  Transform Sensor/LConn1 -- W/RConn1

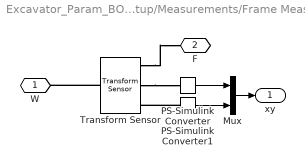
== system Excavator_Param_BOFTOF_Setup/Measurements/Frame Meas11 ==
  Mux : Mux  Inputs=2
  PS-Simulink Converter : nesl_utility/PS-Simulink Converter  PhysicalDomain=network_engine_domain  SubClassName=ps_output  LeftPortType=input  RightPortType=output  PseudoPeriodic=off  Frequencies=[]  VectorFormat=inherit  Unit=inherit  AffineConversion=off
  PS-Simulink Converter1 : nesl_utility/PS-Simulink Converter  PhysicalDomain=network_engine_domain  SubClassName=ps_output  LeftPortType=input  RightPortType=output  PseudoPeriodic=off  Frequencies=[]  VectorFormat=inherit  Unit=inherit  AffineConversion=off
  Transform Sensor : sm_lib/Frames and Transforms/Transform Sensor  MeasurementFrame=World  RotationSequence=XYX  SenseAngle=off  SenseAxis=off  SenseQ=off  SenseR=off  SenseRotationSequence=off  SenseOmegaX=off  SenseOmegaY=off  SenseOmegaZ=off  SenseOmega=off  SenseQDot=off  SenseRDot=off  SenseRotationSequenceDot=off  SenseAlphaX=off  SenseAlphaY=off  SenseAlphaZ=off  SenseAlpha=off  SenseQDDot=off  SenseRDDot=off  SenseX=on  SenseY=on  SenseZ=off  SenseXYZ=off  SenseRad=off  SenseAzim=off  SenseDist=off  SenseInc=off  SenseXDot=off  SenseYDot=off  SenseZDot=off  SenseXYZDot=off  SenseRadDot=off  SenseAzimDot=off  SenseDistDot=off  SenseIncDot=off  SenseXDDot=off  SenseYDDot=off  SenseZDDot=off  SenseXYZDDot=off  SenseRadDDot=off  SenseAzimDDot=off  SenseDistDDot=off  SenseIncDDot=off
  W : PMIOPort  Side=Left
  F : PMIOPort  Port=2  Side=Left
  xy : Outport
  wires:
  PS-Simulink Converter1/1 -> Mux/2
  PS-Simulink Converter/1 -> Mux/1
  Mux/1 -> xy/1
  connections:
  Transform Sensor/LConn1 -- W/RConn1
  Transform Sensor/RConn2 -- PS-Simulink Converter/LConn1
  PS-Simulink Converter1/LConn1 -- Transform Sensor/RConn3
  Transform Sensor/RConn1 -- F/RConn1

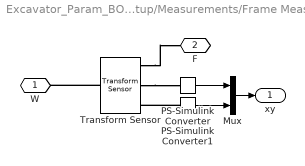
== system Excavator_Param_BOFTOF_Setup/Measurements/Frame Meas12 ==
  Mux : Mux  Inputs=2
  PS-Simulink Converter : nesl_utility/PS-Simulink Converter  PhysicalDomain=network_engine_domain  SubClassName=ps_output  LeftPortType=input  RightPortType=output  PseudoPeriodic=off  Frequencies=[]  VectorFormat=inherit  Unit=inherit  AffineConversion=off
  PS-Simulink Converter1 : nesl_utility/PS-Simulink Converter  PhysicalDomain=network_engine_domain  SubClassName=ps_output  LeftPortType=input  RightPortType=output  PseudoPeriodic=off  Frequencies=[]  VectorFormat=inherit  Unit=inherit  AffineConversion=off
  Transform Sensor : sm_lib/Frames and Transforms/Transform Sensor  MeasurementFrame=World  RotationSequence=XYX  SenseAngle=off  SenseAxis=off  SenseQ=off  SenseR=off  SenseRotationSequence=off  SenseOmegaX=off  SenseOmegaY=off  SenseOmegaZ=off  SenseOmega=off  SenseQDot=off  SenseRDot=off  SenseRotationSequenceDot=off  SenseAlphaX=off  SenseAlphaY=off  SenseAlphaZ=off  SenseAlpha=off  SenseQDDot=off  SenseRDDot=off  SenseX=on  SenseY=on  SenseZ=off  SenseXYZ=off  SenseRad=off  SenseAzim=off  SenseDist=off  SenseInc=off  SenseXDot=off  SenseYDot=off  SenseZDot=off  SenseXYZDot=off  SenseRadDot=off  SenseAzimDot=off  SenseDistDot=off  SenseIncDot=off  SenseXDDot=off  SenseYDDot=off  SenseZDDot=off  SenseXYZDDot=off  SenseRadDDot=off  SenseAzimDDot=off  SenseDistDDot=off  SenseIncDDot=off
  W : PMIOPort  Side=Left
  F : PMIOPort  Port=2  Side=Left
  xy : Outport
  wires:
  Mux/1 -> xy/1
  PS-Simulink Converter/1 -> Mux/1
  PS-Simulink Converter1/1 -> Mux/2
  connections:
  Transform Sensor/RConn1 -- F/RConn1
  PS-Simulink Converter1/LConn1 -- Transform Sensor/RConn3
  Transform Sensor/RConn2 -- PS-Simulink Converter/LConn1
  Transform Sensor/LConn1 -- W/RConn1

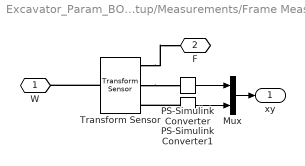
== system Excavator_Param_BOFTOF_Setup/Measurements/Frame Meas13 ==
  Mux : Mux  Inputs=2
  PS-Simulink Converter : nesl_utility/PS-Simulink Converter  PhysicalDomain=network_engine_domain  SubClassName=ps_output  LeftPortType=input  RightPortType=output  PseudoPeriodic=off  Frequencies=[]  VectorFormat=inherit  Unit=inherit  AffineConversion=off
  PS-Simulink Converter1 : nesl_utility/PS-Simulink Converter  PhysicalDomain=network_engine_domain  SubClassName=ps_output  LeftPortType=input  RightPortType=output  PseudoPeriodic=off  Frequencies=[]  VectorFormat=inherit  Unit=inherit  AffineConversion=off
  Transform Sensor : sm_lib/Frames and Transforms/Transform Sensor  MeasurementFrame=World  RotationSequence=XYX  SenseAngle=off  SenseAxis=off  SenseQ=off  SenseR=off  SenseRotationSequence=off  SenseOmegaX=off  SenseOmegaY=off  SenseOmegaZ=off  SenseOmega=off  SenseQDot=off  SenseRDot=off  SenseRotationSequenceDot=off  SenseAlphaX=off  SenseAlphaY=off  SenseAlphaZ=off  SenseAlpha=off  SenseQDDot=off  SenseRDDot=off  SenseX=on  SenseY=on  SenseZ=off  SenseXYZ=off  SenseRad=off  SenseAzim=off  SenseDist=off  SenseInc=off  SenseXDot=off  SenseYDot=off  SenseZDot=off  SenseXYZDot=off  SenseRadDot=off  SenseAzimDot=off  SenseDistDot=off  SenseIncDot=off  SenseXDDot=off  SenseYDDot=off  SenseZDDot=off  SenseXYZDDot=off  SenseRadDDot=off  SenseAzimDDot=off  SenseDistDDot=off  SenseIncDDot=off
  W : PMIOPort  Side=Left
  F : PMIOPort  Port=2  Side=Left
  xy : Outport
  wires:
  PS-Simulink Converter1/1 -> Mux/2
  PS-Simulink Converter/1 -> Mux/1
  Mux/1 -> xy/1
  connections:
  Transform Sensor/LConn1 -- W/RConn1
  Transform Sensor/RConn2 -- PS-Simulink Converter/LConn1
  PS-Simulink Converter1/LConn1 -- Transform Sensor/RConn3
  Transform Sensor/RConn1 -- F/RConn1

== system Excavator_Param_BOFTOF_Setup/Measurements/Frame Meas2 ==
  Mux : Mux  Inputs=2
  PS-Simulink Converter : nesl_utility/PS-Simulink Converter  PhysicalDomain=network_engine_domain  SubClassName=ps_output  LeftPortType=input  RightPortType=output  PseudoPeriodic=off  Frequencies=[]  VectorFormat=inherit  Unit=inherit  AffineConversion=off
  PS-Simulink Converter1 : nesl_utility/PS-Simulink Converter  PhysicalDomain=network_engine_domain  SubClassName=ps_output  LeftPortType=input  RightPortType=output  PseudoPeriodic=off  Frequencies=[]  VectorFormat=inherit  Unit=inherit  AffineConversion=off
  Transform Sensor : sm_lib/Frames and Transforms/Transform Sensor  MeasurementFrame=World  RotationSequence=XYX  SenseAngle=off  SenseAxis=off  SenseQ=off  SenseR=off  SenseRotationSequence=off  SenseOmegaX=off  SenseOmegaY=off  SenseOmegaZ=off  SenseOmega=off  SenseQDot=off  SenseRDot=off  SenseRotationSequenceDot=off  SenseAlphaX=off  SenseAlphaY=off  SenseAlphaZ=off  SenseAlpha=off  SenseQDDot=off  SenseRDDot=off  SenseX=on  SenseY=on  SenseZ=off  SenseXYZ=off  SenseRad=off  SenseAzim=off  SenseDist=off  SenseInc=off  SenseXDot=off  SenseYDot=off  SenseZDot=off  SenseXYZDot=off  SenseRadDot=off  SenseAzimDot=off  SenseDistDot=off  SenseIncDot=off  SenseXDDot=off  SenseYDDot=off  SenseZDDot=off  SenseXYZDDot=off  SenseRadDDot=off  SenseAzimDDot=off  SenseDistDDot=off  SenseIncDDot=off
  W : PMIOPort  Side=Left
  F : PMIOPort  Port=2  Side=Left
  xy : Outport
  wires:
  Mux/1 -> xy/1
  PS-Simulink Converter/1 -> Mux/1
  PS-Simulink Converter1/1 -> Mux/2
  connections:
  Transform Sensor/RConn1 -- F/RConn1
  PS-Simulink Converter1/LConn1 -- Transform Sensor/RConn3
  Transform Sensor/RConn2 -- PS-Simulink Converter/LConn1
  Transform Sensor/LConn1 -- W/RConn1

== system Excavator_Param_BOFTOF_Setup/Measurements/Frame Meas3 ==
  Mux : Mux  Inputs=2
  PS-Simulink Converter : nesl_utility/PS-Simulink Converter  PhysicalDomain=network_engine_domain  SubClassName=ps_output  LeftPortType=input  RightPortType=output  PseudoPeriodic=off  Frequencies=[]  VectorFormat=inherit  Unit=inherit  AffineConversion=off
  PS-Simulink Converter1 : nesl_utility/PS-Simulink Converter  PhysicalDomain=network_engine_domain  SubClassName=ps_output  LeftPortType=input  RightPortType=output  PseudoPeriodic=off  Frequencies=[]  VectorFormat=inherit  Unit=inherit  AffineConversion=off
  Transform Sensor : sm_lib/Frames and Transforms/Transform Sensor  MeasurementFrame=World  RotationSequence=XYX  SenseAngle=off  SenseAxis=off  SenseQ=off  SenseR=off  SenseRotationSequence=off  SenseOmegaX=off  SenseOmegaY=off  SenseOmegaZ=off  SenseOmega=off  SenseQDot=off  SenseRDot=off  SenseRotationSequenceDot=off  SenseAlphaX=off  SenseAlphaY=off  SenseAlphaZ=off  SenseAlpha=off  SenseQDDot=off  SenseRDDot=off  SenseX=on  SenseY=on  SenseZ=off  SenseXYZ=off  SenseRad=off  SenseAzim=off  SenseDist=off  SenseInc=off  SenseXDot=off  SenseYDot=off  SenseZDot=off  SenseXYZDot=off  SenseRadDot=off  SenseAzimDot=off  SenseDistDot=off  SenseIncDot=off  SenseXDDot=off  SenseYDDot=off  SenseZDDot=off  SenseXYZDDot=off  SenseRadDDot=off  SenseAzimDDot=off  SenseDistDDot=off  SenseIncDDot=off
  W : PMIOPort  Side=Left
  F : PMIOPort  Port=2  Side=Left
  xy : Outport
  wires:
  PS-Simulink Converter1/1 -> Mux/2
  PS-Simulink Converter/1 -> Mux/1
  Mux/1 -> xy/1
  connections:
  Transform Sensor/LConn1 -- W/RConn1
  Transform Sensor/RConn2 -- PS-Simulink Converter/LConn1
  PS-Simulink Converter1/LConn1 -- Transform Sensor/RConn3
  Transform Sensor/RConn1 -- F/RConn1

== system Excavator_Param_BOFTOF_Setup/Measurements/Frame Meas4 ==
  Mux : Mux  Inputs=2
  PS-Simulink Converter : nesl_utility/PS-Simulink Converter  PhysicalDomain=network_engine_domain  SubClassName=ps_output  LeftPortType=input  RightPortType=output  PseudoPeriodic=off  Frequencies=[]  VectorFormat=inherit  Unit=inherit  AffineConversion=off
  PS-Simulink Converter1 : nesl_utility/PS-Simulink Converter  PhysicalDomain=network_engine_domain  SubClassName=ps_output  LeftPortType=input  RightPortType=output  PseudoPeriodic=off  Frequencies=[]  VectorFormat=inherit  Unit=inherit  AffineConversion=off
  Transform Sensor : sm_lib/Frames and Transforms/Transform Sensor  MeasurementFrame=World  RotationSequence=XYX  SenseAngle=off  SenseAxis=off  SenseQ=off  SenseR=off  SenseRotationSequence=off  SenseOmegaX=off  SenseOmegaY=off  SenseOmegaZ=off  SenseOmega=off  SenseQDot=off  SenseRDot=off  SenseRotationSequenceDot=off  SenseAlphaX=off  SenseAlphaY=off  SenseAlphaZ=off  SenseAlpha=off  SenseQDDot=off  SenseRDDot=off  SenseX=on  SenseY=on  SenseZ=off  SenseXYZ=off  SenseRad=off  SenseAzim=off  SenseDist=off  SenseInc=off  SenseXDot=off  SenseYDot=off  SenseZDot=off  SenseXYZDot=off  SenseRadDot=off  SenseAzimDot=off  SenseDistDot=off  SenseIncDot=off  SenseXDDot=off  SenseYDDot=off  SenseZDDot=off  SenseXYZDDot=off  SenseRadDDot=off  SenseAzimDDot=off  SenseDistDDot=off  SenseIncDDot=off
  W : PMIOPort  Side=Left
  F : PMIOPort  Port=2  Side=Left
  xy : Outport
  wires:
  Mux/1 -> xy/1
  PS-Simulink Converter/1 -> Mux/1
  PS-Simulink Converter1/1 -> Mux/2
  connections:
  Transform Sensor/RConn1 -- F/RConn1
  PS-Simulink Converter1/LConn1 -- Transform Sensor/RConn3
  Transform Sensor/RConn2 -- PS-Simulink Converter/LConn1
  Transform Sensor/LConn1 -- W/RConn1
